simulink model "testGyrostellar_KF"  (R2021a)
settings: Solver=VariableStepAuto  StartTime=0.0  StopTime=100  RelTol=1e-3
libraries: sharedtransform x4
settings Model: Creator=Laura  LastModifiedBy=Laura

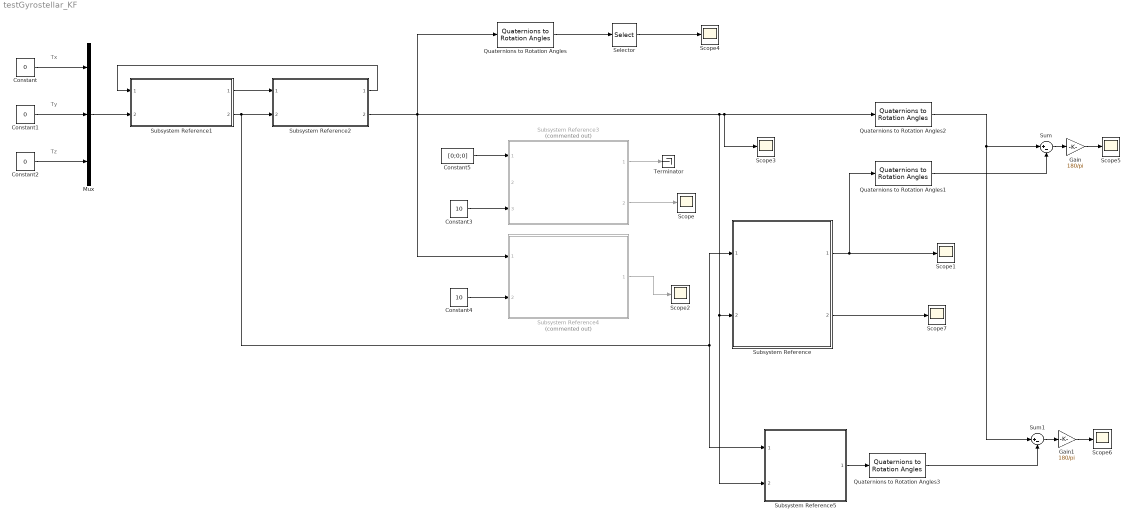
== system testGyrostellar_KF ==
  note: Ty
  note: Tx
  note: Tz
  Constant : Constant  Value=0
  Constant1 : Constant  Value=0
  Constant2 : Constant  Value=0
  Constant3 : Constant  Value=10
  Constant4 : Constant  Value=10
  Constant5 : Constant  Value=[0;0;0]
  Gain : Gain  Gain=180/pi
  Gain1 : Gain  Gain=180/pi
  Mux : Mux  Inputs=3
  Quaternions to Rotation Angles{,1..3} (4 alike) : sharedtransform/Quaternions to Rotation Angles  rotationOrder=ZYX  aMode=aMode
      settings: SourceProductBaseCode=AE,PW,DR,MT,UV,VE
  Scope{,1..7} (8 alike) : Scope
  Selector : Selector  InputPortWidth=3  IndexOptions=Index vector (dialog)  Indices=[1]  OutputSizes=1
  Subsystem Reference : Subsystem  ReferencedSubsystem=Gyrostellar_KF
  Subsystem Reference1 : Subsystem  ReferencedSubsystem=Dynamics
  Subsystem Reference2 : Subsystem  ReferencedSubsystem=Kinematics
  Subsystem Reference3 : Subsystem  Commented=on  ReferencedSubsystem=IMU
  Subsystem Reference4 : Subsystem  Commented=on  ReferencedSubsystem=StarTracker
  Subsystem Reference5 : Subsystem  ReferencedSubsystem=NavigationSolution
  Sum : Sum  Inputs=|+-
  Sum1 : Sum  Inputs=|+-
  Terminator : Terminator
  wires:
  Selector/1 -> Scope4/1
  Subsystem Reference/1 -> Quaternions to Rotation Angles1/1, Scope1/1
  Subsystem Reference3/1 -> Terminator/1
  Subsystem Reference1/2 -> Subsystem Reference/1, Subsystem Reference5/1, Subsystem Reference2/2
  Subsystem Reference2/2 -> Subsystem Reference5/2, Subsystem Reference/2, Quaternions to Rotation Angles2/1, Scope3/1, Subsystem Reference4/1, Quaternions to Rotation Angles/1
  Mux/1 -> Subsystem Reference1/2
  Constant3/1 -> Subsystem Reference3/3
  Constant1/1 -> Mux/2
  Subsystem Reference1/1 -> Subsystem Reference2/1
  Constant/1 -> Mux/1
  Subsystem Reference2/1 -> Subsystem Reference1/1
  Subsystem Reference3/2 -> Scope/1
  Constant4/1 -> Subsystem Reference4/2
  Quaternions to Rotation Angles/1 -> Selector/1
  Constant5/1 -> Subsystem Reference3/1
  Constant2/1 -> Mux/3
  Subsystem Reference4/1 -> Scope2/1
  Subsystem Reference/2 -> Scope7/1
  Quaternions to Rotation Angles2/1 -> Sum1/1, Sum/1
  Quaternions to Rotation Angles1/1 -> Sum/2
  Sum/1 -> Gain/1
  Gain/1 -> Scope5/1
  Subsystem Reference5/1 -> Quaternions to Rotation Angles3/1
  Gain1/1 -> Scope6/1
  Quaternions to Rotation Angles3/1 -> Sum1/2
  Sum1/1 -> Gain1/1
